simulink model "iff_sim"  (R2019b)
settings: Solver=VariableStepAuto  StartTime=0.0  StopTime=T  FixedStep=0.001  MaxStep=0.01  RelTol=1e-3
values from neighbouring files (symbols this model uses):
  bsc = 17    [model_data.m]
  d_r = 0.01*ones(6,1)    [model_data.m]
  Fi_b_z = [0;2/3;4/3;1/3;3/3;5/3]*pi    [model_data.m]
  gain_iff = 0    [linearize_plant.m]    (also in model_data.m = 65)
  ka = 11.86e6    (= 11860000)    [model_data.m]
  ksc = 1.79e5    (= 179000)    [model_data.m]
  l_r = 0.36*ones(6,1)    [model_data.m]
  la00 = 61e-3    (= 0.061)    [model_data.m]
  linderiv = 1    [linearize_plant.m]    (also in model_data.m = 0)
  O_lb = [0;0;0;0;0;0]    [model_data.m]
  q_d = [0.523598775598 0.523598775598 -0.713724378945 0.125327831168 0.281034901503 -0.675131532937 0.281034901503 -0.675131532937 0.523598775598 0.523598775598 -0.713724378945 0.125327831168 ... (12582 elements, 18x699)]    [ik.mat]
  qt_d = [0 0 0 0 0 0 0 0 0 0 0 0 ... (12582 elements, 18x699)]    [ik.mat]
  qtt_d = [6.28830321148e-13 -2.00728322852e-12 2.02267832113e-12 3.08516978789e-12 -6.72993285032e-12 -1.57655277981e-14 7.06082029373e-13 -2.74630882455e-12 2.48904434051e-12 -1.77039226713e-12 -3.57348306345e-12 -1.6692908872e-12 ... (12582 elements, 18x699)]    [ik.mat]
  s = out_ctc.s    [ctc_run.m]
  s_0 = s_d(:,:,1)    [ctc_run.m]    (also in iff_run.m)
  t_d = [0 0.01 0.02 0.03 0.04 0.05 0.06 0.07 0.08 0.09 0.1 0.11 ... (699 elements, 1x699)]    [ik.mat]
  ts_noise = 1.6e-4    (= 0.00016)    [model_data.m]
  v_0 = v_d(:,:,1)    [ctc_run.m]    (also in iff_run.m)
  w_lb = 0.195    [model_data.m]
  W_lb = 0.205    [model_data.m]
  w_ub = 0.195    [model_data.m]
  W_ub = 0.205    [model_data.m]
  X = fminsearch(fun,X0,opts)    [iff_diag_altopt.m]    (also in iff_single_altopt.m)
undefined symbols (not defined in the file or in its folder): Kd, Ki, Kp, t_dist, Y, Z
libraries: nesl_utility x281, sm_lib x208, simulink_extras x36, dspindex x30, simulink x12, powerlib_meascontrol x1
(part 14 of 14)

== system iff_sim/High-authority control/CTC/computed torque control/bases + rods/lower base/O_lb -> G_1 ==
  rot z : sm_lib/Frames and Transforms/Rigid Transform  TranslationMethod=None  TranslationStandardOffset=0  TranslationLengthUnit=m  TranslationStandardAxis=+Z  TranslationCartesianOffset=[0 0 0]  TranslationROffset=0  TranslationROffsetUnits=m  TranslationZOffset=0  TranslationZOffsetUnits=m  TranslationThetaOffset=0  TranslationThetaOffsetUnits=deg  RotationMethod=StandardAxis  RotationAngleUnits=rad  RotationStandardAxis=+Z  RotationAngle=Fi_b_z(1)  RotationArbitraryAxis=[0 0 1]  FollAlignAxisA=+X  BaseAlignAxisA=+Y  FollAlignAxisB=+Y  BaseAlignAxisB=+Z  RotationSequenceAxes=FollowerAxes  RotationSequence=XYX  RotationSequenceAngles=[0 0 0]  RotationSequenceAnglesUnits=deg  RotationMatrix=[1 0 0; 0 1 0; 0 0 1]
  trans z : sm_lib/Frames and Transforms/Rigid Transform  TranslationMethod=StandardAxis  TranslationStandardOffset=h_lb  TranslationLengthUnit=m  TranslationStandardAxis=+Z  TranslationCartesianOffset=[0 0 0]  TranslationROffset=0  TranslationROffsetUnits=m  TranslationZOffset=0  TranslationZOffsetUnits=m  TranslationThetaOffset=0  TranslationThetaOffsetUnits=deg  RotationMethod=None  RotationAngleUnits=deg  RotationStandardAxis=+Z  RotationAngle=0.0  RotationArbitraryAxis=[0 0 1]  FollAlignAxisA=+X  BaseAlignAxisA=+Y  FollAlignAxisB=+Y  BaseAlignAxisB=+Z  RotationSequenceAxes=FollowerAxes  RotationSequence=XYX  RotationSequenceAngles=[0 0 0]  RotationSequenceAnglesUnits=deg  RotationMatrix=[1 0 0; 0 1 0; 0 0 1]
  transl y : sm_lib/Frames and Transforms/Rigid Transform  TranslationMethod=StandardAxis  TranslationStandardOffset=w_lb/2  TranslationLengthUnit=m  TranslationStandardAxis=+Y  TranslationCartesianOffset=[0 0 0]  TranslationROffset=0  TranslationROffsetUnits=m  TranslationZOffset=0  TranslationZOffsetUnits=m  TranslationThetaOffset=0  TranslationThetaOffsetUnits=deg  RotationMethod=None  RotationAngleUnits=deg  RotationStandardAxis=+Z  RotationAngle=0.0  RotationArbitraryAxis=[0 0 1]  FollAlignAxisA=+X  BaseAlignAxisA=+Y  FollAlignAxisB=+Y  BaseAlignAxisB=+Z  RotationSequenceAxes=FollowerAxes  RotationSequence=XYX  RotationSequenceAngles=[0 0 0]  RotationSequenceAnglesUnits=deg  RotationMatrix=[1 0 0; 0 1 0; 0 0 1]
  O_lb : PMIOPort  Side=Left
  G_1 : PMIOPort  Port=2  Side=Right
  connections:
  trans z/LConn1 -- O_lb/RConn1
  trans z/RConn1 -- rot z/LConn1
  transl y/LConn1 -- rot z/RConn1
  transl y/RConn1 -- G_1/RConn1

== system iff_sim/High-authority control/CTC/computed torque control/bases + rods/lower base/O_lb -> G_2 ==
  rot z : sm_lib/Frames and Transforms/Rigid Transform  TranslationMethod=None  TranslationStandardOffset=0  TranslationLengthUnit=m  TranslationStandardAxis=+Z  TranslationCartesianOffset=[0 0 0]  TranslationROffset=0  TranslationROffsetUnits=m  TranslationZOffset=0  TranslationZOffsetUnits=m  TranslationThetaOffset=0  TranslationThetaOffsetUnits=deg  RotationMethod=StandardAxis  RotationAngleUnits=rad  RotationStandardAxis=+Z  RotationAngle=Fi_b_z(2)  RotationArbitraryAxis=[0 0 1]  FollAlignAxisA=+X  BaseAlignAxisA=+Y  FollAlignAxisB=+Y  BaseAlignAxisB=+Z  RotationSequenceAxes=FollowerAxes  RotationSequence=XYX  RotationSequenceAngles=[0 0 0]  RotationSequenceAnglesUnits=deg  RotationMatrix=[1 0 0; 0 1 0; 0 0 1]
  trans z : sm_lib/Frames and Transforms/Rigid Transform  TranslationMethod=StandardAxis  TranslationStandardOffset=h_lb  TranslationLengthUnit=m  TranslationStandardAxis=+Z  TranslationCartesianOffset=[0 0 0]  TranslationROffset=0  TranslationROffsetUnits=m  TranslationZOffset=0  TranslationZOffsetUnits=m  TranslationThetaOffset=0  TranslationThetaOffsetUnits=deg  RotationMethod=None  RotationAngleUnits=deg  RotationStandardAxis=+Z  RotationAngle=0.0  RotationArbitraryAxis=[0 0 1]  FollAlignAxisA=+X  BaseAlignAxisA=+Y  FollAlignAxisB=+Y  BaseAlignAxisB=+Z  RotationSequenceAxes=FollowerAxes  RotationSequence=XYX  RotationSequenceAngles=[0 0 0]  RotationSequenceAnglesUnits=deg  RotationMatrix=[1 0 0; 0 1 0; 0 0 1]
  transl y : sm_lib/Frames and Transforms/Rigid Transform  TranslationMethod=StandardAxis  TranslationStandardOffset=w_lb/2  TranslationLengthUnit=m  TranslationStandardAxis=+Y  TranslationCartesianOffset=[0 0 0]  TranslationROffset=0  TranslationROffsetUnits=m  TranslationZOffset=0  TranslationZOffsetUnits=m  TranslationThetaOffset=0  TranslationThetaOffsetUnits=deg  RotationMethod=None  RotationAngleUnits=deg  RotationStandardAxis=+Z  RotationAngle=0.0  RotationArbitraryAxis=[0 0 1]  FollAlignAxisA=+X  BaseAlignAxisA=+Y  FollAlignAxisB=+Y  BaseAlignAxisB=+Z  RotationSequenceAxes=FollowerAxes  RotationSequence=XYX  RotationSequenceAngles=[0 0 0]  RotationSequenceAnglesUnits=deg  RotationMatrix=[1 0 0; 0 1 0; 0 0 1]
  O_lb : PMIOPort  Side=Left
  G_1 : PMIOPort  Port=2  Side=Right
  connections:
  trans z/LConn1 -- O_lb/RConn1
  trans z/RConn1 -- rot z/LConn1
  transl y/LConn1 -- rot z/RConn1
  transl y/RConn1 -- G_1/RConn1

== system iff_sim/High-authority control/CTC/computed torque control/bases + rods/lower base/O_lb -> G_3 ==
  rot z : sm_lib/Frames and Transforms/Rigid Transform  TranslationMethod=None  TranslationStandardOffset=0  TranslationLengthUnit=m  TranslationStandardAxis=+Z  TranslationCartesianOffset=[0 0 0]  TranslationROffset=0  TranslationROffsetUnits=m  TranslationZOffset=0  TranslationZOffsetUnits=m  TranslationThetaOffset=0  TranslationThetaOffsetUnits=deg  RotationMethod=StandardAxis  RotationAngleUnits=rad  RotationStandardAxis=+Z  RotationAngle=Fi_b_z(3)  RotationArbitraryAxis=[0 0 1]  FollAlignAxisA=+X  BaseAlignAxisA=+Y  FollAlignAxisB=+Y  BaseAlignAxisB=+Z  RotationSequenceAxes=FollowerAxes  RotationSequence=XYX  RotationSequenceAngles=[0 0 0]  RotationSequenceAnglesUnits=deg  RotationMatrix=[1 0 0; 0 1 0; 0 0 1]
  trans z : sm_lib/Frames and Transforms/Rigid Transform  TranslationMethod=StandardAxis  TranslationStandardOffset=h_lb  TranslationLengthUnit=m  TranslationStandardAxis=+Z  TranslationCartesianOffset=[0 0 0]  TranslationROffset=0  TranslationROffsetUnits=m  TranslationZOffset=0  TranslationZOffsetUnits=m  TranslationThetaOffset=0  TranslationThetaOffsetUnits=deg  RotationMethod=None  RotationAngleUnits=deg  RotationStandardAxis=+Z  RotationAngle=0.0  RotationArbitraryAxis=[0 0 1]  FollAlignAxisA=+X  BaseAlignAxisA=+Y  FollAlignAxisB=+Y  BaseAlignAxisB=+Z  RotationSequenceAxes=FollowerAxes  RotationSequence=XYX  RotationSequenceAngles=[0 0 0]  RotationSequenceAnglesUnits=deg  RotationMatrix=[1 0 0; 0 1 0; 0 0 1]
  transl y : sm_lib/Frames and Transforms/Rigid Transform  TranslationMethod=StandardAxis  TranslationStandardOffset=w_lb/2  TranslationLengthUnit=m  TranslationStandardAxis=+Y  TranslationCartesianOffset=[0 0 0]  TranslationROffset=0  TranslationROffsetUnits=m  TranslationZOffset=0  TranslationZOffsetUnits=m  TranslationThetaOffset=0  TranslationThetaOffsetUnits=deg  RotationMethod=None  RotationAngleUnits=deg  RotationStandardAxis=+Z  RotationAngle=0.0  RotationArbitraryAxis=[0 0 1]  FollAlignAxisA=+X  BaseAlignAxisA=+Y  FollAlignAxisB=+Y  BaseAlignAxisB=+Z  RotationSequenceAxes=FollowerAxes  RotationSequence=XYX  RotationSequenceAngles=[0 0 0]  RotationSequenceAnglesUnits=deg  RotationMatrix=[1 0 0; 0 1 0; 0 0 1]
  O_lb : PMIOPort  Side=Left
  G_1 : PMIOPort  Port=2  Side=Right
  connections:
  trans z/LConn1 -- O_lb/RConn1
  trans z/RConn1 -- rot z/LConn1
  transl y/LConn1 -- rot z/RConn1
  transl y/RConn1 -- G_1/RConn1

== system iff_sim/High-authority control/CTC/computed torque control/bases + rods/lower base/wf -> O_lb ==
  rot x : sm_lib/Frames and Transforms/Rigid Transform  TranslationMethod=None  TranslationStandardOffset=0  TranslationLengthUnit=m  TranslationStandardAxis=+Z  TranslationCartesianOffset=[0 0 0]  TranslationROffset=0  TranslationROffsetUnits=m  TranslationZOffset=0  TranslationZOffsetUnits=m  TranslationThetaOffset=0  TranslationThetaOffsetUnits=deg  RotationMethod=StandardAxis  RotationAngleUnits=rad  RotationStandardAxis=+X  RotationAngle=O_lb(4,1)  RotationArbitraryAxis=[0 0 1]  FollAlignAxisA=+X  BaseAlignAxisA=+Y  FollAlignAxisB=+Y  BaseAlignAxisB=+Z  RotationSequenceAxes=FollowerAxes  RotationSequence=XYX  RotationSequenceAngles=[0 0 0]  RotationSequenceAnglesUnits=deg  RotationMatrix=[1 0 0; 0 1 0; 0 0 1]
  rot y : sm_lib/Frames and Transforms/Rigid Transform  TranslationMethod=None  TranslationStandardOffset=0  TranslationLengthUnit=m  TranslationStandardAxis=+Z  TranslationCartesianOffset=[0 0 0]  TranslationROffset=0  TranslationROffsetUnits=m  TranslationZOffset=0  TranslationZOffsetUnits=m  TranslationThetaOffset=0  TranslationThetaOffsetUnits=deg  RotationMethod=StandardAxis  RotationAngleUnits=rad  RotationStandardAxis=+Y  RotationAngle=O_lb(5,1)  RotationArbitraryAxis=[0 0 1]  FollAlignAxisA=+X  BaseAlignAxisA=+Y  FollAlignAxisB=+Y  BaseAlignAxisB=+Z  RotationSequenceAxes=FollowerAxes  RotationSequence=XYX  RotationSequenceAngles=[0 0 0]  RotationSequenceAnglesUnits=deg  RotationMatrix=[1 0 0; 0 1 0; 0 0 1]
  rot z : sm_lib/Frames and Transforms/Rigid Transform  TranslationMethod=None  TranslationStandardOffset=0  TranslationLengthUnit=m  TranslationStandardAxis=+Z  TranslationCartesianOffset=[0 0 0]  TranslationROffset=0  TranslationROffsetUnits=m  TranslationZOffset=0  TranslationZOffsetUnits=m  TranslationThetaOffset=0  TranslationThetaOffsetUnits=deg  RotationMethod=StandardAxis  RotationAngleUnits=rad  RotationStandardAxis=+X  RotationAngle=O_lb(6,1)  RotationArbitraryAxis=[0 0 1]  FollAlignAxisA=+X  BaseAlignAxisA=+Y  FollAlignAxisB=+Y  BaseAlignAxisB=+Z  RotationSequenceAxes=FollowerAxes  RotationSequence=XYX  RotationSequenceAngles=[0 0 0]  RotationSequenceAnglesUnits=deg  RotationMatrix=[1 0 0; 0 1 0; 0 0 1]
  transl : sm_lib/Frames and Transforms/Rigid Transform  TranslationMethod=Cartesian  TranslationStandardOffset=0  TranslationLengthUnit=m  TranslationStandardAxis=+Z  TranslationCartesianOffset=O_lb(1:3,1)  TranslationROffset=0  TranslationROffsetUnits=m  TranslationZOffset=0  TranslationZOffsetUnits=m  TranslationThetaOffset=0  TranslationThetaOffsetUnits=deg  RotationMethod=None  RotationAngleUnits=deg  RotationStandardAxis=+Z  RotationAngle=0.0  RotationArbitraryAxis=[0 0 1]  FollAlignAxisA=+X  BaseAlignAxisA=+Y  FollAlignAxisB=+Y  BaseAlignAxisB=+Z  RotationSequenceAxes=FollowerAxes  RotationSequence=XYX  RotationSequenceAngles=[0 0 0]  RotationSequenceAnglesUnits=deg  RotationMatrix=[1 0 0; 0 1 0; 0 0 1]
  wf : PMIOPort  Side=Left
  O_lb : PMIOPort  Port=2  Side=Right
  connections:
  transl/LConn1 -- wf/RConn1
  transl/RConn1 -- rot x/LConn1
  rot x/RConn1 -- rot y/LConn1
  rot y/RConn1 -- rot z/LConn1
  O_lb/RConn1 -- rot z/RConn1

== system iff_sim/High-authority control/CTC/computed torque control/bases + rods/upper base/O_ub -> H_4 ==
  rot z : sm_lib/Frames and Transforms/Rigid Transform  TranslationMethod=None  TranslationStandardOffset=0  TranslationLengthUnit=m  TranslationStandardAxis=+Z  TranslationCartesianOffset=[0 0 0]  TranslationROffset=0  TranslationROffsetUnits=m  TranslationZOffset=0  TranslationZOffsetUnits=m  TranslationThetaOffset=0  TranslationThetaOffsetUnits=deg  RotationMethod=StandardAxis  RotationAngleUnits=rad  RotationStandardAxis=+Z  RotationAngle=Fi_b_z(4)  RotationArbitraryAxis=[0 0 1]  FollAlignAxisA=+X  BaseAlignAxisA=+Y  FollAlignAxisB=+Y  BaseAlignAxisB=+Z  RotationSequenceAxes=FollowerAxes  RotationSequence=XYX  RotationSequenceAngles=[0 0 0]  RotationSequenceAnglesUnits=deg  RotationMatrix=[1 0 0; 0 1 0; 0 0 1]
  trans z : sm_lib/Frames and Transforms/Rigid Transform  TranslationMethod=StandardAxis  TranslationStandardOffset=h_ub  TranslationLengthUnit=m  TranslationStandardAxis=-Z  TranslationCartesianOffset=[0 0 0]  TranslationROffset=0  TranslationROffsetUnits=m  TranslationZOffset=0  TranslationZOffsetUnits=m  TranslationThetaOffset=0  TranslationThetaOffsetUnits=deg  RotationMethod=None  RotationAngleUnits=deg  RotationStandardAxis=+Z  RotationAngle=0.0  RotationArbitraryAxis=[0 0 1]  FollAlignAxisA=+X  BaseAlignAxisA=+Y  FollAlignAxisB=+Y  BaseAlignAxisB=+Z  RotationSequenceAxes=FollowerAxes  RotationSequence=XYX  RotationSequenceAngles=[0 0 0]  RotationSequenceAnglesUnits=deg  RotationMatrix=[1 0 0; 0 1 0; 0 0 1]
  transl y : sm_lib/Frames and Transforms/Rigid Transform  TranslationMethod=StandardAxis  TranslationStandardOffset=w_ub/2  TranslationLengthUnit=m  TranslationStandardAxis=+Y  TranslationCartesianOffset=[0 0 0]  TranslationROffset=0  TranslationROffsetUnits=m  TranslationZOffset=0  TranslationZOffsetUnits=m  TranslationThetaOffset=0  TranslationThetaOffsetUnits=deg  RotationMethod=None  RotationAngleUnits=deg  RotationStandardAxis=+Z  RotationAngle=0.0  RotationArbitraryAxis=[0 0 1]  FollAlignAxisA=+X  BaseAlignAxisA=+Y  FollAlignAxisB=+Y  BaseAlignAxisB=+Z  RotationSequenceAxes=FollowerAxes  RotationSequence=XYX  RotationSequenceAngles=[0 0 0]  RotationSequenceAnglesUnits=deg  RotationMatrix=[1 0 0; 0 1 0; 0 0 1]
  O_ub : PMIOPort  Side=Left
  H_4 : PMIOPort  Port=2  Side=Right
  connections:
  trans z/LConn1 -- O_ub/RConn1
  trans z/RConn1 -- rot z/LConn1
  transl y/LConn1 -- rot z/RConn1
  transl y/RConn1 -- H_4/RConn1

== system iff_sim/High-authority control/CTC/computed torque control/bases + rods/upper base/O_ub -> H_5 ==
  rot z : sm_lib/Frames and Transforms/Rigid Transform  TranslationMethod=None  TranslationStandardOffset=0  TranslationLengthUnit=m  TranslationStandardAxis=+Z  TranslationCartesianOffset=[0 0 0]  TranslationROffset=0  TranslationROffsetUnits=m  TranslationZOffset=0  TranslationZOffsetUnits=m  TranslationThetaOffset=0  TranslationThetaOffsetUnits=deg  RotationMethod=StandardAxis  RotationAngleUnits=rad  RotationStandardAxis=+Z  RotationAngle=Fi_b_z(5)  RotationArbitraryAxis=[0 0 1]  FollAlignAxisA=+X  BaseAlignAxisA=+Y  FollAlignAxisB=+Y  BaseAlignAxisB=+Z  RotationSequenceAxes=FollowerAxes  RotationSequence=XYX  RotationSequenceAngles=[0 0 0]  RotationSequenceAnglesUnits=deg  RotationMatrix=[1 0 0; 0 1 0; 0 0 1]
  trans z : sm_lib/Frames and Transforms/Rigid Transform  TranslationMethod=StandardAxis  TranslationStandardOffset=h_ub  TranslationLengthUnit=m  TranslationStandardAxis=-Z  TranslationCartesianOffset=[0 0 0]  TranslationROffset=0  TranslationROffsetUnits=m  TranslationZOffset=0  TranslationZOffsetUnits=m  TranslationThetaOffset=0  TranslationThetaOffsetUnits=deg  RotationMethod=None  RotationAngleUnits=deg  RotationStandardAxis=+Z  RotationAngle=0.0  RotationArbitraryAxis=[0 0 1]  FollAlignAxisA=+X  BaseAlignAxisA=+Y  FollAlignAxisB=+Y  BaseAlignAxisB=+Z  RotationSequenceAxes=FollowerAxes  RotationSequence=XYX  RotationSequenceAngles=[0 0 0]  RotationSequenceAnglesUnits=deg  RotationMatrix=[1 0 0; 0 1 0; 0 0 1]
  transl y : sm_lib/Frames and Transforms/Rigid Transform  TranslationMethod=StandardAxis  TranslationStandardOffset=w_ub/2  TranslationLengthUnit=m  TranslationStandardAxis=+Y  TranslationCartesianOffset=[0 0 0]  TranslationROffset=0  TranslationROffsetUnits=m  TranslationZOffset=0  TranslationZOffsetUnits=m  TranslationThetaOffset=0  TranslationThetaOffsetUnits=deg  RotationMethod=None  RotationAngleUnits=deg  RotationStandardAxis=+Z  RotationAngle=0.0  RotationArbitraryAxis=[0 0 1]  FollAlignAxisA=+X  BaseAlignAxisA=+Y  FollAlignAxisB=+Y  BaseAlignAxisB=+Z  RotationSequenceAxes=FollowerAxes  RotationSequence=XYX  RotationSequenceAngles=[0 0 0]  RotationSequenceAnglesUnits=deg  RotationMatrix=[1 0 0; 0 1 0; 0 0 1]
  O_ub : PMIOPort  Side=Left
  H_5 : PMIOPort  Port=2  Side=Right
  connections:
  trans z/LConn1 -- O_ub/RConn1
  trans z/RConn1 -- rot z/LConn1
  transl y/LConn1 -- rot z/RConn1
  transl y/RConn1 -- H_5/RConn1

== system iff_sim/High-authority control/CTC/computed torque control/bases + rods/upper base/O_ub -> H_6 ==
  rot z : sm_lib/Frames and Transforms/Rigid Transform  TranslationMethod=None  TranslationStandardOffset=0  TranslationLengthUnit=m  TranslationStandardAxis=+Z  TranslationCartesianOffset=[0 0 0]  TranslationROffset=0  TranslationROffsetUnits=m  TranslationZOffset=0  TranslationZOffsetUnits=m  TranslationThetaOffset=0  TranslationThetaOffsetUnits=deg  RotationMethod=StandardAxis  RotationAngleUnits=rad  RotationStandardAxis=+Z  RotationAngle=Fi_b_z(6)  RotationArbitraryAxis=[0 0 1]  FollAlignAxisA=+X  BaseAlignAxisA=+Y  FollAlignAxisB=+Y  BaseAlignAxisB=+Z  RotationSequenceAxes=FollowerAxes  RotationSequence=XYX  RotationSequenceAngles=[0 0 0]  RotationSequenceAnglesUnits=deg  RotationMatrix=[1 0 0; 0 1 0; 0 0 1]
  trans z : sm_lib/Frames and Transforms/Rigid Transform  TranslationMethod=StandardAxis  TranslationStandardOffset=h_ub  TranslationLengthUnit=m  TranslationStandardAxis=-Z  TranslationCartesianOffset=[0 0 0]  TranslationROffset=0  TranslationROffsetUnits=m  TranslationZOffset=0  TranslationZOffsetUnits=m  TranslationThetaOffset=0  TranslationThetaOffsetUnits=deg  RotationMethod=None  RotationAngleUnits=deg  RotationStandardAxis=+Z  RotationAngle=0.0  RotationArbitraryAxis=[0 0 1]  FollAlignAxisA=+X  BaseAlignAxisA=+Y  FollAlignAxisB=+Y  BaseAlignAxisB=+Z  RotationSequenceAxes=FollowerAxes  RotationSequence=XYX  RotationSequenceAngles=[0 0 0]  RotationSequenceAnglesUnits=deg  RotationMatrix=[1 0 0; 0 1 0; 0 0 1]
  transl y : sm_lib/Frames and Transforms/Rigid Transform  TranslationMethod=StandardAxis  TranslationStandardOffset=w_ub/2  TranslationLengthUnit=m  TranslationStandardAxis=+Y  TranslationCartesianOffset=[0 0 0]  TranslationROffset=0  TranslationROffsetUnits=m  TranslationZOffset=0  TranslationZOffsetUnits=m  TranslationThetaOffset=0  TranslationThetaOffsetUnits=deg  RotationMethod=None  RotationAngleUnits=deg  RotationStandardAxis=+Z  RotationAngle=0.0  RotationArbitraryAxis=[0 0 1]  FollAlignAxisA=+X  BaseAlignAxisA=+Y  FollAlignAxisB=+Y  BaseAlignAxisB=+Z  RotationSequenceAxes=FollowerAxes  RotationSequence=XYX  RotationSequenceAngles=[0 0 0]  RotationSequenceAnglesUnits=deg  RotationMatrix=[1 0 0; 0 1 0; 0 0 1]
  O_ub : PMIOPort  Side=Left
  H_6 : PMIOPort  Port=2  Side=Right
  connections:
  trans z/LConn1 -- O_ub/RConn1
  trans z/RConn1 -- rot z/LConn1
  transl y/LConn1 -- rot z/RConn1
  transl y/RConn1 -- H_6/RConn1

== matlab function iff_sim/High-authority control/CTC/computed torque control/bases + rods/v_r,v_ub -> v ==
  data: v_1 input; v output; v_2 input; v_3 input; v_4 input; v_5 input; v_6 input; v_ub input
function v = fcn(v_1,v_2,v_3,v_4,v_5,v_6,v_ub)
    v = [v_1,v_2,v_3,v_4,v_5,v_6,v_ub];
end

== matlab function iff_sim/dynamic model/v -> qt ==
  data: v input; qt output
function qt = fcn(v)
    qt = zeros(18,1);
    for r = 1:1:6
        qt(((r-1)*2+1):((r-1)*2+2),1) = v(4:5,r);
    end
    qt(13:end) = v(:,7);
end

== matlab function iff_sim/High-authority control/CTC/computed torque control/desired cable vectors// lengths/cable 2/cable force and length ==
  data: pz input; F_c output; fz input; l_c output
function [F_c,l_c] = fcn(pz,fz)
    if pz < 0 
        F_c = fz;
    else
        F_c = -fz;
    end
    l_c = abs(pz);
end

== matlab function iff_sim/dynamic model/rods + bases/s_r,s_ub -> s ==
  data: s_1 input; s output; s_2 input; s_3 input; s_4 input; s_5 input; s_6 input; s_ub input
function s = fcn(s_1,s_2,s_3,s_4,s_5,s_6,s_ub)
    s = [s_1,s_2,s_3,s_4,s_5,s_6,s_ub];
end

== matlab function iff_sim/dynamic model/rods + bases/v_r,v_ub -> v ==
  data: v_1 input; v output; v_2 input; v_3 input; v_4 input; v_5 input; v_6 input; v_ub input
function v = fcn(v_1,v_2,v_3,v_4,v_5,v_6,v_ub)
    v = [v_1,v_2,v_3,v_4,v_5,v_6,v_ub];
end

== matlab function iff_sim/High-authority control/CTC/computed torque control/desired cable vectors// lengths/cable 1/cable force and length ==
  data: pz input; F_c output; fz input; l_c output
function [F_c,l_c] = fcn(pz,fz)
    if pz < 0 
        F_c = fz;
    else
        F_c = -fz;
    end
    l_c = abs(pz);
end

== matlab function iff_sim/High-authority control/CTC/computed torque control/desired cable vectors// lengths/cable 3/cable force and length ==
  data: pz input; F_c output; fz input; l_c output
function [F_c,l_c] = fcn(pz,fz)
    if pz < 0 
        F_c = fz;
    else
        F_c = -fz;
    end
    l_c = abs(pz);
end

== matlab function iff_sim/High-authority control/CTC/computed torque control/desired cable vectors// lengths/cable 4/cable force and length ==
  data: pz input; F_c output; fz input; l_c output
function [F_c,l_c] = fcn(pz,fz)
    if pz < 0 
        F_c = fz;
    else
        F_c = -fz;
    end
    l_c = abs(pz);
end

== matlab function iff_sim/High-authority control/CTC/computed torque control/desired cable vectors// lengths/cable 5/cable force and length ==
  data: pz input; F_c output; fz input; l_c output
function [F_c,l_c] = fcn(pz,fz)
    if pz < 0 
        F_c = fz;
    else
        F_c = -fz;
    end
    l_c = abs(pz);
end

== matlab function iff_sim/High-authority control/CTC/computed torque control/desired cable vectors// lengths/cable 6/cable force and length ==
  data: pz input; F_c output; fz input; l_c output
function [F_c,l_c] = fcn(pz,fz)
    if pz < 0 
        F_c = fz;
    else
        F_c = -fz;
    end
    l_c = abs(pz);
end

== matlab function iff_sim/High-authority control/CTC/computed torque control/desired cable vectors// lengths/cable 7/cable force and length ==
  data: pz input; F_c output; fz input; l_c output
function [F_c,l_c] = fcn(pz,fz)
    if pz < 0 
        F_c = fz;
    else
        F_c = -fz;
    end
    l_c = abs(pz);
end

== matlab function iff_sim/High-authority control/CTC/computed torque control/desired cable vectors// lengths/cable 8/cable force and length ==
  data: pz input; F_c output; fz input; l_c output
function [F_c,l_c] = fcn(pz,fz)
    if pz < 0 
        F_c = fz;
    else
        F_c = -fz;
    end
    l_c = abs(pz);
end

== matlab function iff_sim/High-authority control/CTC/computed torque control/desired cable vectors// lengths/cable 9/cable force and length ==
  data: pz input; F_c output; fz input; l_c output
function [F_c,l_c] = fcn(pz,fz)
    if pz < 0 
        F_c = fz;
    else
        F_c = -fz;
    end
    l_c = abs(pz);
end

== matlab function iff_sim/High-authority control/CTC/computed torque control/desired cable vectors// lengths/cable 10/cable force and length ==
  data: pz input; F_c output; fz input; l_c output
function [F_c,l_c] = fcn(pz,fz)
    if pz < 0 
        F_c = fz;
    else
        F_c = -fz;
    end
    l_c = abs(pz);
end

== matlab function iff_sim/High-authority control/CTC/computed torque control/desired cable vectors// lengths/cable 11/cable force and length ==
  data: pz input; F_c output; fz input; l_c output
function [F_c,l_c] = fcn(pz,fz)
    if pz < 0 
        F_c = fz;
    else
        F_c = -fz;
    end
    l_c = abs(pz);
end

== matlab function iff_sim/High-authority control/CTC/computed torque control/desired cable vectors// lengths/cable 12/cable force and length ==
  data: pz input; F_c output; fz input; l_c output
function [F_c,l_c] = fcn(pz,fz)
    if pz < 0 
        F_c = fz;
    else
        F_c = -fz;
    end
    l_c = abs(pz);
end

== matlab function iff_sim/High-authority control/CTC/computed torque control/desired cable vectors// lengths/cable 13/cable force and length ==
  data: pz input; F_c output; fz input; l_c output
function [F_c,l_c] = fcn(pz,fz)
    if pz < 0 
        F_c = fz;
    else
        F_c = -fz;
    end
    l_c = abs(pz);
end

== matlab function iff_sim/High-authority control/CTC/computed torque control/desired cable vectors// lengths/cable 14/cable force and length ==
  data: pz input; F_c output; fz input; l_c output
function [F_c,l_c] = fcn(pz,fz)
    if pz < 0 
        F_c = fz;
    else
        F_c = -fz;
    end
    l_c = abs(pz);
end

== matlab function iff_sim/High-authority control/CTC/computed torque control/desired cable vectors// lengths/cable 15/cable force and length ==
  data: pz input; F_c output; fz input; l_c output
function [F_c,l_c] = fcn(pz,fz)
    if pz < 0 
        F_c = fz;
    else
        F_c = -fz;
    end
    l_c = abs(pz);
end

== matlab function iff_sim/High-authority control/CTC/computed torque control/desired cable vectors// lengths/cable 16/cable force and length ==
  data: pz input; F_c output; fz input; l_c output
function [F_c,l_c] = fcn(pz,fz)
    if pz < 0 
        F_c = fz;
    else
        F_c = -fz;
    end
    l_c = abs(pz);
end

== matlab function iff_sim/High-authority control/CTC/computed torque control/bases + rods/s_r,s_ub -> s ==
  data: s_1 input; s output; s_2 input; s_3 input; s_4 input; s_5 input; s_6 input; s_ub input
function s = fcn(s_1,s_2,s_3,s_4,s_5,s_6,s_ub)
    s = [s_1,s_2,s_3,s_4,s_5,s_6,s_ub];
end

== matlab function iff_sim/High-authority control/CTC/computed torque control/desired cable vectors// lengths/cable 17/cable force and length ==
  data: pz input; F_c output; fz input; l_c output
function [F_c,l_c] = fcn(pz,fz)
    if pz < 0 
        F_c = fz;
    else
        F_c = -fz;
    end
    l_c = abs(pz);
end

== matlab function iff_sim/dynamic model/s -> q ==
  data: s input; q output
function q = fcn(s)
    q = zeros(18,1);
    for r = 1:1:6
        q(((r-1)*2+1):((r-1)*2+2),1) = s(4:5,r);
    end
    q(13:end) = s(:,7);
end

== matlab function iff_sim/High-authority control/CTC/computed torque control/desired cable vectors// lengths/cable 18/cable force and length ==
  data: pz input; F_c output; fz input; l_c output
function [F_c,l_c] = fcn(pz,fz)
    if pz < 0 
        F_c = fz;
    else
        F_c = -fz;
    end
    l_c = abs(pz);
end
